simulink model "rocketsim"  (R2018a)
settings: Solver=FixedStepAuto  StartTime=0.0  StopTime=250  EnableMultiTasking=on
undefined symbols (not defined in the file): A_e, area, C_A_0, C_A_alpha, C_A_beta, C_Mp_alpha, C_Mp_q, C_Mr_0, C_Mr_p, C_My_beta, C_My_r, C_N_0, C_N_alpha, C_S_0, C_S_beta, dotm, Earth, engines, J, l, m, minv, omega_E, omegaJ, p_e, r_gim, r_init, rotZ, t_burn, v_e, WGS84
libraries: aerolibtransform2 x3, aerolibutil x3, aerolibatmos2 x1, aerolibgravity2 x1, sharedutil x1, simulink_extras x1
settings Model: Creator=Matyas  LastModifiedBy=hrist
settings DataIOCC: ExternalInput=[0 0 0 0 0 0]  InitialState=[]  LimitDataPoints=on  LoadExternalInput=on  LoadInitialState=on  SaveFormat=StructureWithTime
settings OptimizationCC: DefaultParameterBehavior=Inlined  BufferReuse=off  LifeSpan=inf
settings DebuggingCC: AllowSymbolicDim=off  InitInArrayFormatMsg=none  SFUnexpectedBacktrackingDiag=warning  SFNoUnconditionalDefaultTransitionDiag=warning  SFExecutionAtInitializationDiag=none
settings ModelReferenceCC: PropagateSignalLabelsOutOfModel=off
settings CodeAppCC: StateflowObjectComments=on
settings GRTTargetCC: TargetLangStandard=C89/C90 (ANSI)
settings ConfigComp: CovMetricSettings=dw  CovHtmlReporting=on  CovSaveCumulativeToWorkspaceVar=on  CovSaveSingleToWorkspaceVar=on  CovExternalEMLEnable=off

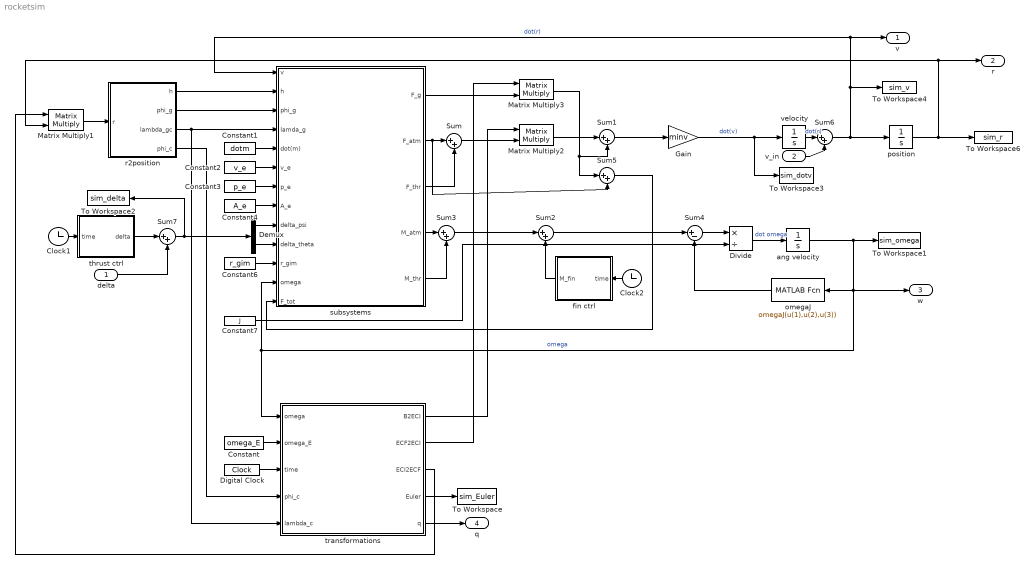
== system rocketsim ==
  delta : Inport  PortDimensions=2
  v_in : Inport  Port=2  PortDimensions=3
  Clock1 : Clock
  Clock2 : Clock
  Constant : Constant  Value=omega_E
  Constant1 : Constant  Value=dotm
  Constant2 : Constant  Value=v_e
  Constant3 : Constant  Value=p_e
  Constant4 : Constant  Value=A_e
  Constant6 : Constant  Value=r_gim
  Constant7 : Constant  Value=J  VectorParams1D=off
  Demux : Demux  Outputs=2
  Digital Clock : DigitalClock
  Divide : Product  Inputs=*/
  Gain : Gain  Gain=minv
  Matrix Multiply1 : Product  Multiplication=Matrix(*)
  Matrix Multiply2 : Product  Multiplication=Matrix(*)
  Matrix Multiply3 : Product  Multiplication=Matrix(*)
  Sum{,1..3,5..7} (7 alike) : Sum  Inputs=|++
  Sum4 : Sum  Inputs=|+-
  To Workspace : ToWorkspace  VariableName=sim_Euler  SaveFormat=Structure With Time  SampleTime=-1
  To Workspace1 : ToWorkspace  VariableName=sim_omega  SaveFormat=Structure With Time  SampleTime=-1
  To Workspace2 : ToWorkspace  VariableName=sim_delta  SaveFormat=Structure With Time  SampleTime=-1
  To Workspace3 : ToWorkspace  VariableName=sim_dotv  SaveFormat=Structure With Time  SampleTime=-1
  To Workspace4 : ToWorkspace  VariableName=sim_v  SaveFormat=Structure With Time  SampleTime=-1
  To Workspace6 : ToWorkspace  VariableName=sim_r  SaveFormat=Structure With Time  SampleTime=-1
  ang velocity : Integrator  InitialCondition=[0; 0; 0]
  fin ctrl : MATLAB Function  TreatAsAtomicUnit=on
  omegaJ : MATLABFcn  MATLABFcn=omegaJ(u(1),u(2),u(3))
  position : Integrator  InitialCondition=r_init
  r2position : Subsystem
  subsystems : Subsystem
  thrust ctrl : MATLAB Function  TreatAsAtomicUnit=on
  transformations : Subsystem
  velocity : Integrator  InitialCondition=[600 0 0]
  v : Outport
  r : Outport  Port=2
  w : Outport  Port=3
  q : Outport  Port=4
  wires:
  position/1 -> r/1, Matrix Multiply1/2, To Workspace6/1
  Constant/1 -> transformations/2(omega_E)
  Constant1/1 -> subsystems/5(dot(m))
  Constant2/1 -> subsystems/6(v_e)
  Constant3/1 -> subsystems/7(p_e)
  Constant4/1 -> subsystems/8(A_e)
  subsystems/2(F_atm) -> Sum5/2, Sum/1
  subsystems/3(F_thr) -> Sum/2
  Matrix Multiply2/1 -> Sum1/1
  Sum1/1 -> Gain/1
  Gain/1 -> To Workspace3/1, velocity/1  "dot(v)"
  Sum6/1 -> subsystems/1(v), v/1, To Workspace4/1, position/1  "dot(r)"
  Constant6/1 -> subsystems/11(r_gim)
  ang velocity/1 -> To Workspace1/1, omegaJ/1, subsystems/12(omega), transformations/1(omega), w/1  "omega"
  Divide/1 -> ang velocity/1  "dot omega"
  Sum4/1 -> Divide/1
  Constant7/1 -> Divide/2
  Sum/1 -> Matrix Multiply2/2
  r2position/1(h) -> subsystems/2(h)
  r2position/2(phi_g) -> subsystems/3(phi_g)
  r2position/3(lambda_gc) -> transformations/5(lambda_c), subsystems/4(lamda_g)
  Digital Clock/1 -> transformations/3(time)
  r2position/4(phi_c) -> transformations/4(phi_c)
  transformations/1(B2ECI) -> Matrix Multiply2/1
  transformations/4(Euler) -> To Workspace/1
  Clock1/1 -> thrust ctrl/1(time)
  thrust ctrl/1(delta) -> Sum7/1
  fin ctrl/1(M_fin) -> Sum2/2
  Clock2/1 -> fin ctrl/1(time)
  Sum2/1 -> Sum4/1
  Sum3/1 -> Sum2/1
  omegaJ/1 -> Sum4/2
  transformations/3(ECI2ECF) -> Matrix Multiply1/1
  transformations/2(ECF2ECI) -> Matrix Multiply3/1
  subsystems/5(M_thr) -> Sum3/2
  Demux/1 -> subsystems/9(delta_psi)
  Demux/2 -> subsystems/10(delta_theta)
  subsystems/4(M_atm) -> Sum3/1
  transformations/5(q) -> q/1
  subsystems/1(F_g) -> Matrix Multiply3/2
  Matrix Multiply3/1 -> Sum5/1, Sum1/2
  Matrix Multiply1/1 -> r2position/1(r)
  Sum5/1 -> subsystems/13(F_tot)
  velocity/1 -> Sum6/1  "dot(r)"
  v_in/1 -> Sum6/2
  delta/1 -> Sum7/2
  Sum7/1 -> To Workspace2/1, Demux/1

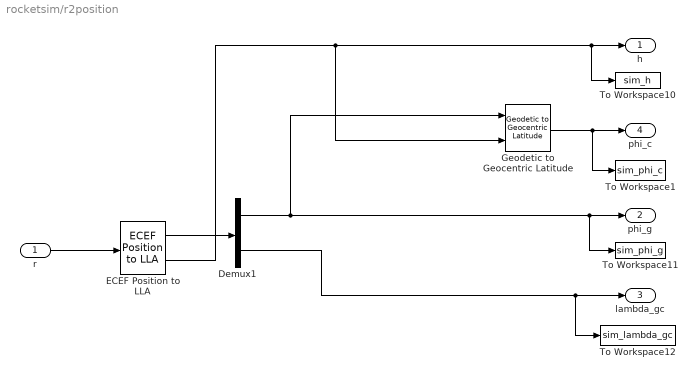
== system rocketsim/r2position ==
  r : Inport
  Demux1 : Demux  Outputs=2
  ECEF Position to LLA : aerolibtransform2/ECEF Position to LLA  units=Metric (MKS)  ptype=Earth (WGS84)  F=1/298.257223563  R=6378137
      settings: SourceProductName=Aerospace Blockset  SourceProductBaseCode=AE
  Geodetic to Geocentric Latitude : aerolibtransform2/Geodetic to  Geocentric Latitude  units=Metric (MKS)  ptype=Earth (WGS84)  F=1/298.257223563  R=6378137  wraplatitude=on
      settings: SourceProductName=Aerospace Blockset  SourceProductBaseCode=AE
  To Workspace1 : ToWorkspace  VariableName=sim_phi_c  SaveFormat=Structure With Time  SampleTime=-1
  To Workspace10 : ToWorkspace  VariableName=sim_h  SaveFormat=Structure With Time  SampleTime=-1
  To Workspace11 : ToWorkspace  VariableName=sim_phi_g  SaveFormat=Structure With Time  SampleTime=-1
  To Workspace12 : ToWorkspace  VariableName=sim_lambda_gc  SaveFormat=Structure With Time  SampleTime=-1
  h : Outport
  phi_g : Outport  Port=2
  lambda_gc : Outport  Port=3
  phi_c : Outport  Port=4
  wires:
  r/1 -> ECEF Position to LLA/1
  ECEF Position to LLA/1 -> Demux1/1
  ECEF Position to LLA/2 -> Geodetic to Geocentric Latitude/2, To Workspace10/1, h/1
  Demux1/1 -> To Workspace11/1, phi_g/1, Geodetic to Geocentric Latitude/1
  Demux1/2 -> lambda_gc/1, To Workspace12/1
  Geodetic to Geocentric Latitude/1 -> To Workspace1/1, phi_c/1

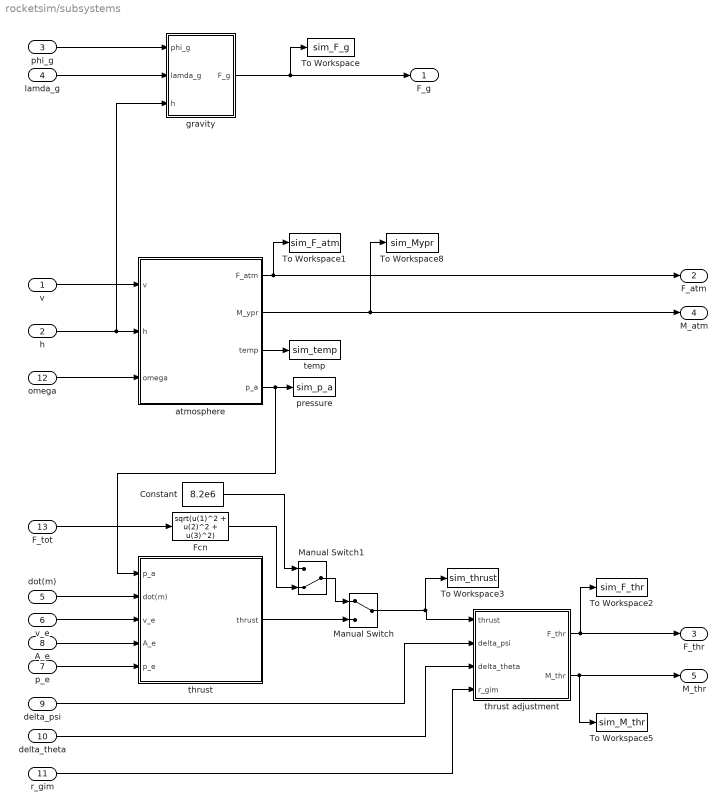
== system rocketsim/subsystems ==
  v : Inport
  h : Inport  Port=2
  phi_g : Inport  Port=3
  lamda_g : Inport  Port=4
  dot(m) : Inport  Port=5
  v_e : Inport  Port=6
  p_e : Inport  Port=7
  A_e : Inport  Port=8
  delta_psi : Inport  Port=9
  delta_theta : Inport  Port=10
  r_gim : Inport  Port=11
  omega : Inport  Port=12
  F_tot : Inport  Port=13
  Constant : Constant  Value=8.2e6
  Fcn : Fcn  Expr=sqrt(u(1)^2 + u(2)^2 + u(3)^2)
  Manual Switch : ManualSwitch
  Manual Switch1 : ManualSwitch  CurrentSetting=0
  To Workspace : ToWorkspace  VariableName=sim_F_g  SaveFormat=Structure With Time  SampleTime=-1
  To Workspace1 : ToWorkspace  VariableName=sim_F_atm  SaveFormat=Structure With Time  SampleTime=-1
  To Workspace2 : ToWorkspace  VariableName=sim_F_thr  SaveFormat=Structure With Time  SampleTime=-1
  To Workspace3 : ToWorkspace  VariableName=sim_thrust  SaveFormat=Structure With Time  SampleTime=-1
  To Workspace5 : ToWorkspace  VariableName=sim_M_thr  SaveFormat=Structure With Time  SampleTime=-1
  To Workspace8 : ToWorkspace  VariableName=sim_Mypr  SaveFormat=Structure With Time  SampleTime=-1
  atmosphere : Subsystem
  gravity : Subsystem
  pressure : ToWorkspace  VariableName=sim_p_a  SaveFormat=Structure With Time  SampleTime=-1
  temp : ToWorkspace  VariableName=sim_temp  SaveFormat=Structure With Time  SampleTime=-1
  thrust : Subsystem
  thrust adjustment : Subsystem
  F_g : Outport
  F_atm : Outport  Port=2
  F_thr : Outport  Port=3
  M_atm : Outport  Port=4
  M_thr : Outport  Port=5
  wires:
  phi_g/1 -> gravity/1(phi_g)
  lamda_g/1 -> gravity/2(lamda_g)
  h/1 -> atmosphere/2(h), gravity/3(h)
  v/1 -> atmosphere/1(v)
  atmosphere/4(p_a) -> pressure/1, thrust/1(p_a)
  v_e/1 -> thrust/3(v_e)
  p_e/1 -> thrust/5(p_e)
  A_e/1 -> thrust/4(A_e)
  dot(m)/1 -> thrust/2(dot(m))
  atmosphere/3(temp) -> temp/1
  atmosphere/1(F_atm) -> F_atm/1, To Workspace1/1
  atmosphere/2(M_ypr) -> M_atm/1, To Workspace8/1
  gravity/1(F_g) -> To Workspace/1, F_g/1
  thrust adjustment/1(F_thr) -> To Workspace2/1, F_thr/1
  delta_psi/1 -> thrust adjustment/2(delta_psi)
  delta_theta/1 -> thrust adjustment/3(delta_theta)
  r_gim/1 -> thrust adjustment/4(r_gim)
  thrust adjustment/2(M_thr) -> To Workspace5/1, M_thr/1
  omega/1 -> atmosphere/3(omega)
  F_tot/1 -> Fcn/1
  Manual Switch/1 -> To Workspace3/1, thrust adjustment/1(thrust)
  thrust/1(thrust) -> Manual Switch/2
  Manual Switch1/1 -> Manual Switch/1
  Constant/1 -> Manual Switch1/1
  Fcn/1 -> Manual Switch1/2

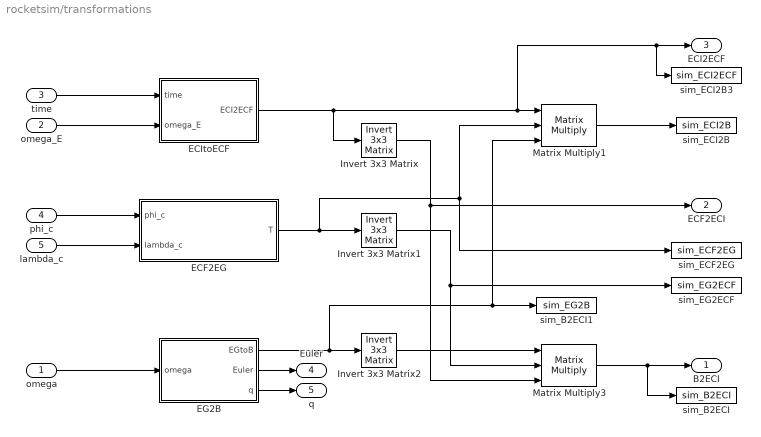
== system rocketsim/transformations ==
  omega : Inport
  omega_E : Inport  Port=2
  time : Inport  Port=3
  phi_c : Inport  Port=4
  lambda_c : Inport  Port=5
  ECF2EG : MATLAB Function  TreatAsAtomicUnit=on
  ECItoECF : Subsystem
  EG2B : Subsystem
  Invert 3x3 Matrix : aerolibutil/Invert  3x3 Matrix
  Invert 3x3 Matrix1 : aerolibutil/Invert  3x3 Matrix
  Invert 3x3 Matrix2 : aerolibutil/Invert  3x3 Matrix
  Matrix Multiply1 : Product  Inputs=3  Multiplication=Matrix(*)
  Matrix Multiply3 : Product  Inputs=3  Multiplication=Matrix(*)
  sim_B2ECI : ToWorkspace  VariableName=sim_B2ECI  SaveFormat=Structure With Time  SampleTime=-1
  sim_B2ECI1 : ToWorkspace  VariableName=sim_EG2B  SaveFormat=Structure With Time  SampleTime=-1
  sim_ECF2EG : ToWorkspace  VariableName=sim_ECF2EG  SaveFormat=Structure With Time  SampleTime=-1
  sim_ECI2B : ToWorkspace  VariableName=sim_ECI2B  SaveFormat=Structure With Time  SampleTime=-1
  sim_ECI2B3 : ToWorkspace  VariableName=sim_ECI2ECF  SaveFormat=Structure With Time  SampleTime=-1
  sim_EG2ECF : ToWorkspace  VariableName=sim_EG2ECF  SaveFormat=Structure With Time  SampleTime=-1
  B2ECI : Outport
  ECF2ECI : Outport  Port=2
  ECI2ECF : Outport  Port=3
  Euler : Outport  Port=4
  q : Outport  Port=5
  wires:
  omega/1 -> EG2B/1(omega)
  omega_E/1 -> ECItoECF/2(omega_E)
  time/1 -> ECItoECF/1(time)
  phi_c/1 -> ECF2EG/1(phi_c)
  lambda_c/1 -> ECF2EG/2(lambda_c)
  ECItoECF/1(ECI2ECF) -> sim_ECI2B3/1, ECI2ECF/1, Matrix Multiply1/1, Invert 3x3 Matrix/1
  ECF2EG/1(T) -> Matrix Multiply1/2, sim_ECF2EG/1, Invert 3x3 Matrix1/1
  Invert 3x3 Matrix2/1 -> Matrix Multiply3/1
  Invert 3x3 Matrix1/1 -> sim_EG2ECF/1, Matrix Multiply3/2
  Matrix Multiply3/1 -> B2ECI/1, sim_B2ECI/1
  Matrix Multiply1/1 -> sim_ECI2B/1
  EG2B/2(Euler) -> Euler/1
  Invert 3x3 Matrix/1 -> Matrix Multiply3/3, ECF2ECI/1
  EG2B/1(EGtoB) -> Matrix Multiply1/3, sim_B2ECI1/1, Invert 3x3 Matrix2/1
  EG2B/3(q) -> q/1

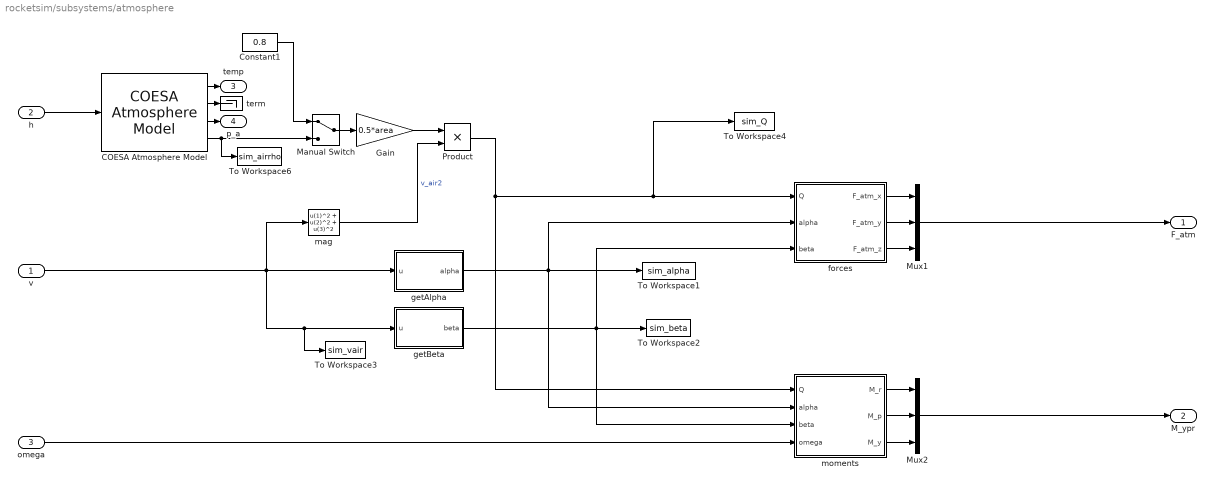
== system rocketsim/subsystems/atmosphere ==
  v : Inport
  h : Inport  Port=2
  omega : Inport  Port=3
  COESA Atmosphere Model : aerolibatmos2/COESA Atmosphere Model  units=Metric (MKS)  spec=1976 COESA-extended U.S. Standard Atmosphere  model=Profile  profile_var=High temperature  profile_percent=1%  profile_alt=5 km (16404 ft)  envelope_var=High temperature  envelope_percent=1%  action=Warning
  Constant1 : Constant  Value=0.8
  Gain : Gain  Gain=0.5*area
  Manual Switch : ManualSwitch
  Mux1 : Mux  Inputs=3
  Mux2 : Mux  Inputs=3
  Product : Product
  To Workspace1 : ToWorkspace  VariableName=sim_alpha  SaveFormat=Structure With Time  SampleTime=-1
  To Workspace2 : ToWorkspace  VariableName=sim_beta  SaveFormat=Structure With Time  SampleTime=-1
  To Workspace3 : ToWorkspace  VariableName=sim_vair  SaveFormat=Structure With Time  SampleTime=-1
  To Workspace4 : ToWorkspace  VariableName=sim_Q  SaveFormat=Structure With Time  SampleTime=-1
  To Workspace6 : ToWorkspace  VariableName=sim_airrho  SaveFormat=Structure With Time  SampleTime=-1
  forces : Subsystem
  getAlpha : MATLAB Function  TreatAsAtomicUnit=on
  getBeta : MATLAB Function  TreatAsAtomicUnit=on
  mag : Fcn  Expr=u(1)^2 + u(2)^2 + u(3)^2
  moments : Subsystem
  term : Terminator
  F_atm : Outport
  M_ypr : Outport  Port=2
  temp : Outport  Port=3
  p_a : Outport  Port=4
  wires:
  COESA Atmosphere Model/2 -> term/1
  COESA Atmosphere Model/1 -> temp/1
  COESA Atmosphere Model/3 -> p_a/1
  COESA Atmosphere Model/4 -> To Workspace6/1, Manual Switch/2
  Product/1 -> moments/1(Q), To Workspace4/1, forces/1(Q)
  h/1 -> COESA Atmosphere Model/1
  mag/1 -> Product/2  "v_air2"
  getAlpha/1(alpha) -> To Workspace1/1, forces/2(alpha), moments/2(alpha)
  getBeta/1(beta) -> To Workspace2/1, forces/3(beta), moments/3(beta)
  forces/1(F_atm_x) -> Mux1/1
  forces/2(F_atm_y) -> Mux1/2
  forces/3(F_atm_z) -> Mux1/3
  Mux1/1 -> F_atm/1
  moments/1(M_r) -> Mux2/1
  moments/2(M_p) -> Mux2/2
  moments/3(M_y) -> Mux2/3
  Mux2/1 -> M_ypr/1
  v/1 -> To Workspace3/1, getBeta/1(u), getAlpha/1(u), mag/1
  omega/1 -> moments/4(omega)
  Gain/1 -> Product/1
  Manual Switch/1 -> Gain/1
  Constant1/1 -> Manual Switch/1

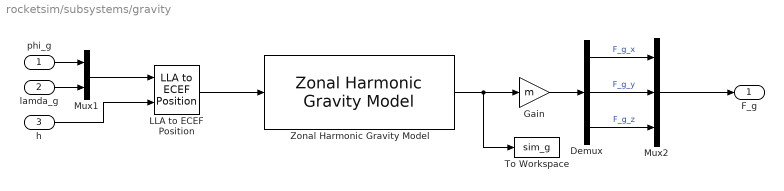
== system rocketsim/subsystems/gravity ==
  phi_g : Inport
  lamda_g : Inport  Port=2
  h : Inport  Port=3
  Demux : Demux  Outputs=3
  Gain : Gain  Gain=m
  LLA to ECEF Position : aerolibtransform2/LLA to ECEF Position  units=Metric (MKS)  ptype=Earth (WGS84)  F=1/298.257223563  R=6378137
      settings: SourceProductName=Aerospace Blockset  SourceProductBaseCode=AE
  Mux1 : Mux  Inputs=2
  Mux2 : Mux  Inputs=3
  To Workspace : ToWorkspace  VariableName=sim_g  SaveFormat=Structure With Time  SampleTime=-1
  Zonal Harmonic Gravity Model : aerolibgravity2/Zonal Harmonic Gravity Model  units=Metric (MKS)  degree=4  action=Warning  ptype=Earth  R=6378136.3  GM=398600441500000  jvalue=[1.0826269e-03 -2.5323000e-06 -1.6204000e-06]
      settings: SourceProductName=Aerospace Blockset  SourceProductBaseCode=AE
  F_g : Outport
  wires:
  phi_g/1 -> Mux1/1
  lamda_g/1 -> Mux1/2
  Gain/1 -> Demux/1
  Demux/1 -> Mux2/1  "F_g_x"
  Demux/2 -> Mux2/2  "F_g_y"
  Demux/3 -> Mux2/3  "F_g_z"
  LLA to ECEF Position/1 -> Zonal Harmonic Gravity Model/1
  Mux1/1 -> LLA to ECEF Position/1
  h/1 -> LLA to ECEF Position/2
  Zonal Harmonic Gravity Model/1 -> Gain/1, To Workspace/1
  Mux2/1 -> F_g/1

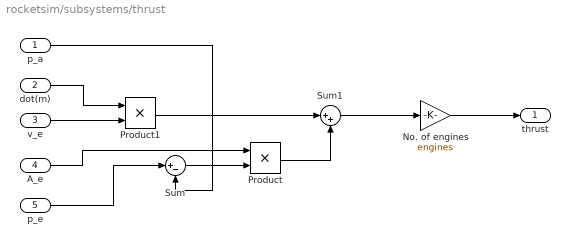
== system rocketsim/subsystems/thrust ==
  p_a : Inport
  dot(m) : Inport  Port=2
  v_e : Inport  Port=3
  A_e : Inport  Port=4
  p_e : Inport  Port=5
  No. of engines : Gain  Gain=engines
  Product : Product
  Product1 : Product
  Sum : Sum  Inputs=|+-
  Sum1 : Sum  Inputs=|++
  thrust : Outport
  wires:
  p_e/1 -> Sum/1
  A_e/1 -> Product/1
  v_e/1 -> Product1/2
  p_a/1 -> Sum/2
  Sum/1 -> Product/2
  Product1/1 -> Sum1/1
  dot(m)/1 -> Product1/1
  Product/1 -> Sum1/2
  No. of engines/1 -> thrust/1
  Sum1/1 -> No. of engines/1

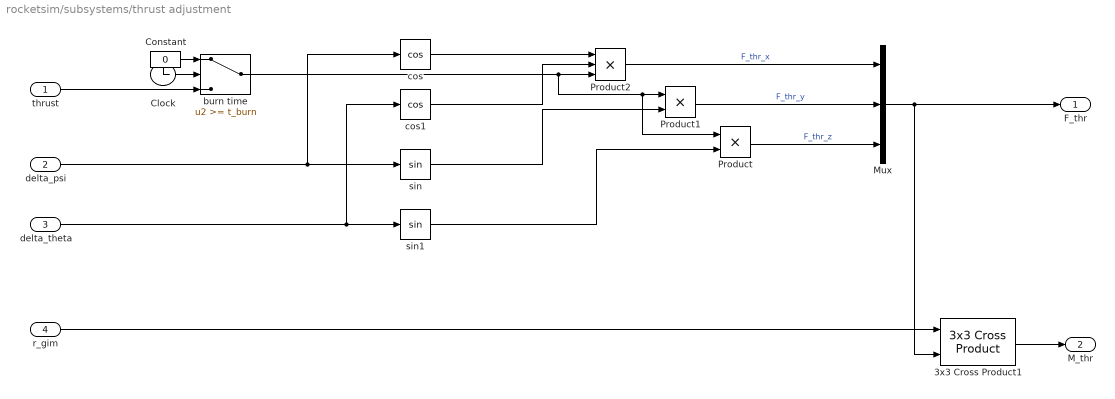
== system rocketsim/subsystems/thrust adjustment ==
  thrust : Inport
  delta_psi : Inport  Port=2
  delta_theta : Inport  Port=3
  r_gim : Inport  Port=4
  3x3 Cross Product1 : sharedutil/3x3 Cross Product  aMode=aMode
      settings: SourceProductBaseCode=AE
  Clock : Clock
  Constant : Constant  Value=0
  Mux : Mux  Inputs=3
  Product : Product
  Product1 : Product
  Product2 : Product  Inputs=3
  burn time : Switch  Threshold=t_burn
  cos : Trigonometry  Operator=cos
  cos1 : Trigonometry  Operator=cos
  sin : Trigonometry
  sin1 : Trigonometry
  F_thr : Outport
  M_thr : Outport  Port=2
  wires:
  sin/1 -> Product1/2
  cos/1 -> Product2/1
  delta_theta/1 -> sin1/1, cos1/1
  cos1/1 -> Product2/2
  Mux/1 -> 3x3 Cross Product1/2, F_thr/1
  thrust/1 -> burn time/3
  Clock/1 -> burn time/2
  delta_psi/1 -> sin/1, cos/1
  sin1/1 -> Product/2
  Product2/1 -> Mux/1  "F_thr_x"
  Product1/1 -> Mux/2  "F_thr_y"
  Product/1 -> Mux/3  "F_thr_z"
  burn time/1 -> Product/1, Product1/1, Product2/3
  3x3 Cross Product1/1 -> M_thr/1
  r_gim/1 -> 3x3 Cross Product1/1
  Constant/1 -> burn time/1

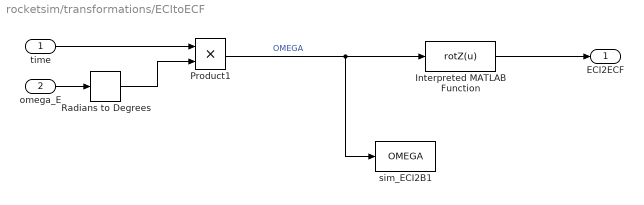
== system rocketsim/transformations/ECItoECF ==
  time : Inport
  omega_E : Inport  Port=2
  Interpreted MATLAB Function : MATLABFcn  MATLABFcn=rotZ(u)  Output1D=off
  Product1 : Product
  Radians to Degrees : simulink_extras/Transformations/Radians to Degrees
  sim_ECI2B1 : ToWorkspace  VariableName=OMEGA  SaveFormat=Structure With Time  SampleTime=-1
  ECI2ECF : Outport
  wires:
  time/1 -> Product1/1
  Interpreted MATLAB Function/1 -> ECI2ECF/1
  Product1/1 -> sim_ECI2B1/1, Interpreted MATLAB Function/1  "OMEGA"
  omega_E/1 -> Radians to Degrees/1
  Radians to Degrees/1 -> Product1/2

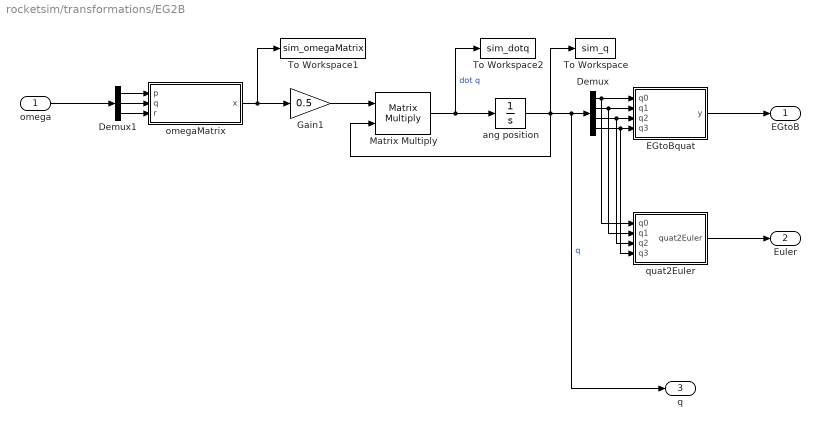
== system rocketsim/transformations/EG2B ==
  omega : Inport
  Demux : Demux
  Demux1 : Demux  Outputs=3
  EGtoBquat : MATLAB Function  TreatAsAtomicUnit=on
  Gain1 : Gain  Gain=0.5
  Matrix Multiply : Product  Multiplication=Matrix(*)
  To Workspace : ToWorkspace  VariableName=sim_q  SaveFormat=Structure With Time  SampleTime=-1
  To Workspace1 : ToWorkspace  VariableName=sim_omegaMatrix  SaveFormat=Structure With Time  SampleTime=-1
  To Workspace2 : ToWorkspace  VariableName=sim_dotq  SaveFormat=Structure With Time  SampleTime=-1
  ang position : Integrator  InitialCondition=[1; 0; 0; 0]
  omegaMatrix : MATLAB Function  TreatAsAtomicUnit=on
  quat2Euler : MATLAB Function  TreatAsAtomicUnit=on
  EGtoB : Outport
  Euler : Outport  Port=2
  q : Outport  Port=3
  wires:
  ang position/1 -> To Workspace/1, q/1, Demux/1, Matrix Multiply/2  "q"
  Demux1/3 -> omegaMatrix/3(r)
  Matrix Multiply/1 -> To Workspace2/1, ang position/1  "dot q"
  Demux1/2 -> omegaMatrix/2(q)
  Demux/3 -> quat2Euler/3(q2), EGtoBquat/3(q2)
  omegaMatrix/1(x) -> To Workspace1/1, Gain1/1
  Demux/1 -> quat2Euler/1(q0), EGtoBquat/1(q0)
  Demux1/1 -> omegaMatrix/1(p)
  Gain1/1 -> Matrix Multiply/1
  Demux/2 -> quat2Euler/2(q1), EGtoBquat/2(q1)
  Demux/4 -> quat2Euler/4(q3), EGtoBquat/4(q3)
  omega/1 -> Demux1/1
  EGtoBquat/1(y) -> EGtoB/1
  quat2Euler/1(quat2Euler) -> Euler/1

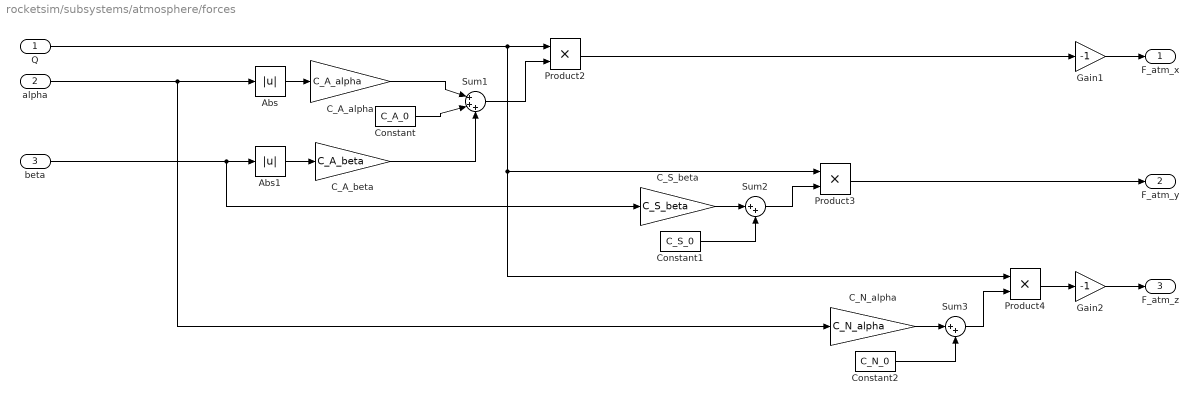
== system rocketsim/subsystems/atmosphere/forces ==
  Q : Inport
  alpha : Inport  Port=2
  beta : Inport  Port=3
  Abs : Abs
  Abs1 : Abs
  C_A_alpha : Gain  Gain=C_A_alpha
  C_A_beta : Gain  Gain=C_A_beta
  C_N_alpha : Gain  Gain=C_N_alpha
  C_S_beta : Gain  Gain=C_S_beta
  Constant : Constant  Value=C_A_0
  Constant1 : Constant  Value=C_S_0
  Constant2 : Constant  Value=C_N_0
  Gain1 : Gain  Gain=-1
  Gain2 : Gain  Gain=-1
  Product2 : Product
  Product3 : Product
  Product4 : Product
  Sum1 : Sum  Inputs=|+++
  Sum2 : Sum  Inputs=|++
  Sum3 : Sum  Inputs=|++
  F_atm_x : Outport
  F_atm_y : Outport  Port=2
  F_atm_z : Outport  Port=3
  wires:
  Product2/1 -> Gain1/1
  Sum2/1 -> Product3/2
  C_N_alpha/1 -> Sum3/1
  Constant1/1 -> Sum2/2
  Constant2/1 -> Sum3/2
  Sum3/1 -> Product4/2
  Product4/1 -> Gain2/1
  Sum1/1 -> Product2/2
  Gain1/1 -> F_atm_x/1
  Constant/1 -> Sum1/2
  C_S_beta/1 -> Sum2/1
  Product3/1 -> F_atm_y/1
  Gain2/1 -> F_atm_z/1
  C_A_alpha/1 -> Sum1/1
  C_A_beta/1 -> Sum1/3
  beta/1 -> Abs1/1, C_S_beta/1
  Q/1 -> Product2/1, Product4/1, Product3/1
  alpha/1 -> Abs/1, C_N_alpha/1
  Abs/1 -> C_A_alpha/1
  Abs1/1 -> C_A_beta/1

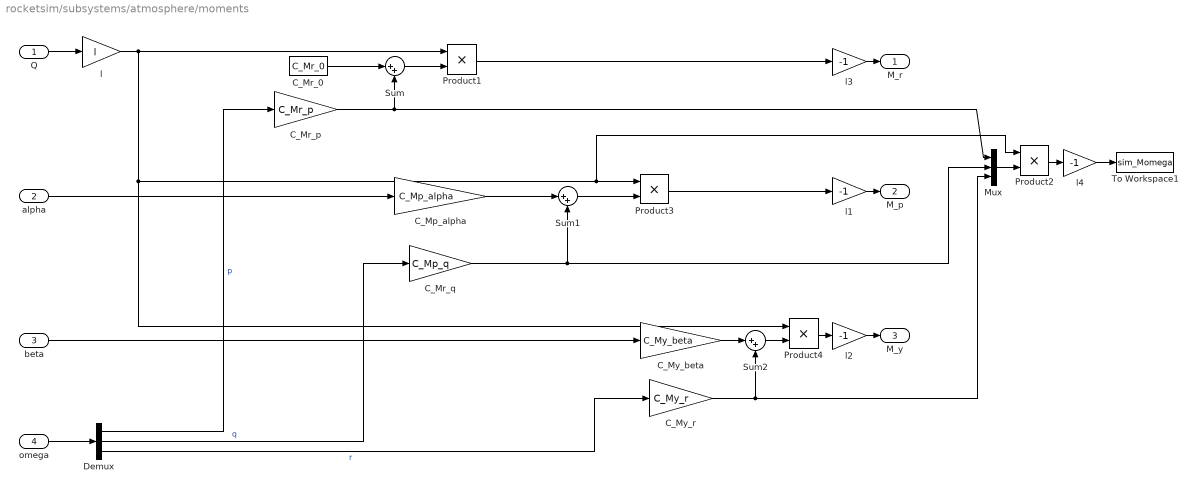
== system rocketsim/subsystems/atmosphere/moments ==
  Q : Inport
  alpha : Inport  Port=2
  beta : Inport  Port=3
  omega : Inport  Port=4
  C_Mp_alpha : Gain  Gain=C_Mp_alpha
  C_Mr_0 : Constant  Value=C_Mr_0
  C_Mr_p : Gain  Gain=C_Mr_p
  C_Mr_q : Gain  Gain=C_Mp_q
  C_My_beta : Gain  Gain=C_My_beta
  C_My_r : Gain  Gain=C_My_r
  Demux : Demux  Outputs=3
  Mux : Mux  Inputs=3
  Product{1..4} (4 alike) : Product
  Sum : Sum  Inputs=|++
  Sum1 : Sum  Inputs=|++
  Sum2 : Sum  Inputs=|++
  To Workspace1 : ToWorkspace  VariableName=sim_Momega  SaveFormat=Structure With Time  SampleTime=-1
  l : Gain  Gain=l
  l{1..4} (4 alike) : Gain  Gain=-1
  M_r : Outport
  M_p : Outport  Port=2
  M_y : Outport  Port=3
  wires:
  alpha/1 -> C_Mp_alpha/1
  l/1 -> Product4/1, Product2/1, Product3/1, Product1/1
  beta/1 -> C_My_beta/1
  Q/1 -> l/1
  l1/1 -> M_p/1
  l2/1 -> M_y/1
  C_Mr_0/1 -> Sum/1
  C_Mr_p/1 -> Sum/2, Mux/1
  Product3/1 -> l1/1
  C_Mr_q/1 -> Sum1/2, Mux/2
  Product4/1 -> l2/1
  C_My_r/1 -> Sum2/2, Mux/3
  omega/1 -> Demux/1
  Demux/1 -> C_Mr_p/1  "p"
  Demux/2 -> C_Mr_q/1  "q"
  Demux/3 -> C_My_r/1  "r"
  Sum/1 -> Product1/2
  C_Mp_alpha/1 -> Sum1/1
  Sum1/1 -> Product3/2
  C_My_beta/1 -> Sum2/1
  Sum2/1 -> Product4/2
  Mux/1 -> Product2/2
  l3/1 -> M_r/1
  Product1/1 -> l3/1
  Product2/1 -> l4/1
  l4/1 -> To Workspace1/1

== matlab function rocketsim/transformations/EG2B/omegaMatrix ==
  data: p input; x output; q input; r input
%% Creates matrix from equation 2.13
function x  = omegaMatrix(p, q, r)
    x = [0 -p -q -r;
         p 0 r -q;
         q -r 0 p;
         r q -p 0];
end

== matlab function rocketsim/transformations/EG2B/EGtoBquat ==
  data: q0 input; y output; q1 input; q2 input; q3 input
%% Transformation quaternion matrix from EG to B
function y = u(q0, q1, q2, q3)
    y = [q0^2 + q1^2 - q2^2 - q3^2, 2*q1*q2 - 2*q0*q3,          2*q0*q2 + 2*q1*q3;
         2*q0*q3 + 2*q1*q2,         q0^2 - q1^2 + q2^2 - q3^2,  2*q2*q3 - 2*q0*q1;
         2*q1*q3 - 2*q0*q2,         2*q0*q1 + 2*q2*q3,          q0^2 - q1^2 - q2^2 + q3^2];
end

== matlab function rocketsim/transformations/ECF2EG ==
  data: phi_c input; T output; lambda_c input
%% Transformation matrix from ECF to EG
function T = ECF2EG(phi_c, lambda_c)
    T = rotY(-phi_c)*rotZ(lambda_c);
end

== matlab function rocketsim/transformations/EG2B/quat2Euler ==
  data: q0 input; quat2Euler output; q1 input; q2 input; q3 input
%% Returns Euler angles from quaternions.
function quat2Euler = u(q0, q1, q2, q3)
    newphi = atan(2*(q2*q3+q0*q1)/(q0^2 - q1^2 - q2^2 + q3^2));
    newtheta = asin(2*(q0*q2 - q1*q3));
    newpsi = atan(2*(q1*q2+q0*q3)/(q0^2 + q1^2 - q2^2 - q3^2));
    
    quat2Euler = [newphi; newtheta; newpsi];
end

== matlab function rocketsim/fin ctrl ==
  data: time input; M_fin output double size=3
%% Fin control
% Values for angles should be from the interval (1,10)

function M_fin = fcn(time)
      
    M_A = [0;0;0];
    M_B = [0;0;0];
    M_C = [0;0;0];
    M_D = [0;0;0];
            
%     if (time > 40 && time < 41)
%         M_B = tiltFin('B', 5);
%         M_D = tiltFin('D', 5);
%     end
    
%     if (time > 100 && time < 101)
%         M_B = tiltFin('B', -2);
%         M_D = tiltFin('D', -2);
%     end
%      
%     if (time > 90 && time < 91)
%         M_A = tiltFin('A', +4);
%         M_C = tiltFin('C', +4);
%     end
        
M_fin = M_A + M_B + M_C + M_D;  

%% Fin control manual

% A (+) & C (-) -> CW from above (+roll)
% A (-) & C (+) -> ACW from above (-roll)
% A & C (+) -> deflecting from Z axis (-pitch)
% A & C (-) -> tilting towards Z axis (+pitch)

% B (+) & D (-) -> ACW from above (-roll)
% B (-) & D (+) -> CW from above (+roll)
% B & D (+) -> deflecting from Y axis (+yaw)
% B & D (-) -> tilting towards Y axis (-yaw)

== matlab function rocketsim/thrust ctrl ==
  data: time input; delta output double
%% Thrust vectoring control
% Values for delta should be of the 10^(-4) order

function delta = fcn(time)

    delta_theta = 0;
    delta_psi = 0;
                
%     if (time > 20 && time < 40)
%         delta_theta = 5e-4;
%     end
     
%     if (time > 30 && time < 100)
%        delta_psi = -5e-4;
%     end

    delta = [delta_psi; delta_theta];        
end

== matlab function rocketsim/subsystems/atmosphere/getBeta ==
  data: u input; beta output
function beta = getBeta(u)
    beta = 0;
    if (u(1) ~= 0)
        %beta = - asin(u(2) / sqrt(u(1)^2 + u(2)^2 + u(3)^2));
        beta = - atan2d(u(2),u(1));
    end
    if abs(beta) < 1e-5
        beta = 0;
    end
end

== matlab function rocketsim/subsystems/atmosphere/getAlpha ==
  data: u input; alpha output
function alpha = getAlpha(u)
    alpha = 0;
    if (u(1) ~= 0)
        alpha = atan2d(u(3), u(1));
    end
%     if abs(alpha) < 1e-5
%         alpha = 0;
%     end
end
